simulink model "src_2022b"  (R2022b)
settings: Solver=VariableStepAuto  StartTime=0.0  StopTime=10.0  RelTol=1e-3
libraries: simulink x2, dspsrcs4 x1
settings Model: Creator=padlewsk  LastModifiedBy=padlewsk
settings OptimizationCC: ReuseModelBlockBuffer=on

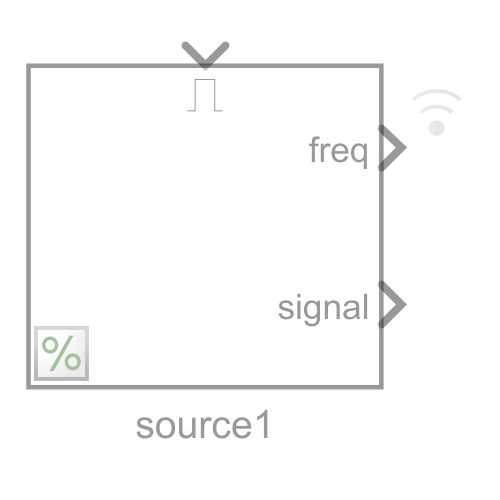
[thumbnail: Simulink's stored preview of the top-level diagram]
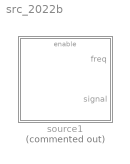
== system src_2022b ==
  source1 : Subsystem  Commented=on  TreatAsAtomicUnit=on

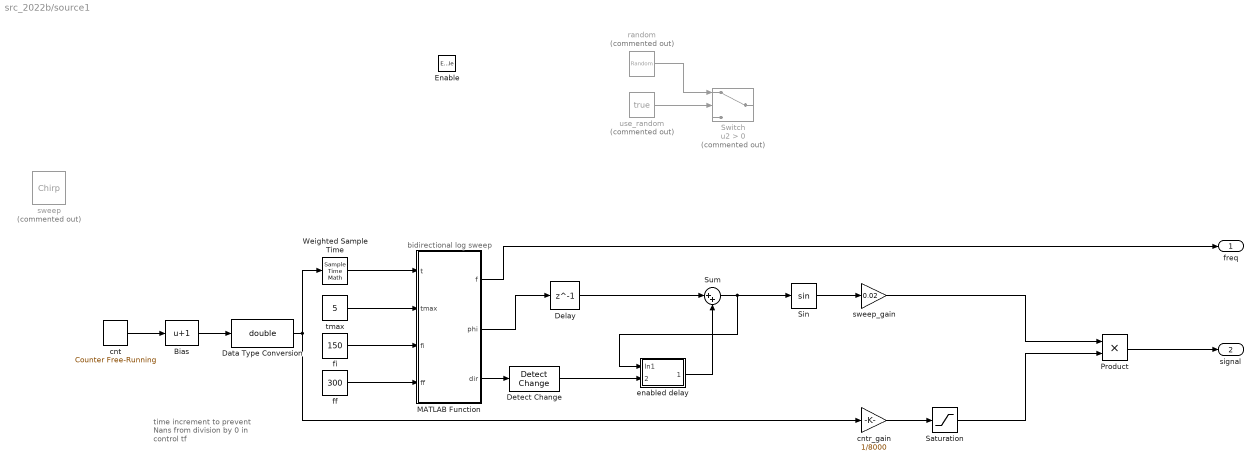
== system src_2022b/source1 ==
  note: bidirectional log sweep
  note: time increment to prevent Nans from division by 0 in control tf
  Enable : EnablePort  StatesWhenEnabling=reset
  Bias : Bias  Bias=1  SaturateOnIntegerOverflow=off
  Data Type Conversion : DataTypeConversion  OutDataTypeStr=double  SaturateOnIntegerOverflow=off  RndMeth=Floor
  Delay : Delay  DelayLength=1
  Detect Change : simulink/Logic and Bit Operations/Detect Change  vinit=false  OutDataTypeStr=boolean
  MATLAB Function : MATLAB Function  TreatAsAtomicUnit=on
  Product : Product
  Saturation : Saturate  UpperLimit=1  LowerLimit=0
  Sin : Trigonometry
  Sum : Sum  Inputs=|++
  Switch : Switch  Commented=on  Criteria=u2 > Threshold  SaturateOnIntegerOverflow=off  InputSameDT=off
  Weighted Sample Time : SampleTimeMath  TsampMathOp=*
  cnt : simulink/Sources/Counter Free-Running  NumBits=32  tsamp=-1
  cntr_gain : Gain  Gain=1/8000  ParamDataTypeStr=double
  enabled delay : Subsystem
  ff : Constant  Value=300
  fi : Constant  Value=150
  random : RandomNumber  Commented=on  Variance=0.5  SampleTime=3.5e-05
  sweep : dspsrcs4/Chirp  Commented=on  sweep=Logarithmic  mode=Bidirectional  f0=150  f1=1200  t1=10  Tsweep=20  phase=0  Ts=3.5e-05  spf=1  datatype=Double  OutputFrames=off
  sweep_gain : Gain  Gain=0.02
  tmax : Constant  Value=5
  use_random : Constant  Commented=on  Value=true  SampleTime=-1
  freq : Outport  OutputWhenDisabled=reset  InitialOutput=0  VectorParamsAs1DForOutWhenUnconnected=off
  signal : Outport  Port=2  OutputWhenDisabled=reset  InitialOutput=0  VectorParamsAs1DForOutWhenUnconnected=off
  wires:
  use_random/1 -> Switch/2
  random/1 -> Switch/1
  sweep_gain/1 -> Product/1
  cntr_gain/1 -> Saturation/1
  Product/1 -> signal/1
  MATLAB Function/2(phi) -> Delay/1
  Saturation/1 -> Product/2
  Weighted Sample Time/1 -> MATLAB Function/1(t)
  Data Type Conversion/1 -> cntr_gain/1, Weighted Sample Time/1
  MATLAB Function/1(f) -> freq/1
  Sin/1 -> sweep_gain/1
  MATLAB Function/3(dir) -> Detect Change/1
  Detect Change/1 -> enabled delay/2(enable)
  Delay/1 -> Sum/1
  enabled delay/1(Out1) -> Sum/2
  Sum/1 -> enabled delay/1(In1), Sin/1
  cnt/1 -> Bias/1
  Bias/1 -> Data Type Conversion/1
  ff/1 -> MATLAB Function/4(ff)
  tmax/1 -> MATLAB Function/2(tmax)
  fi/1 -> MATLAB Function/3(fi)

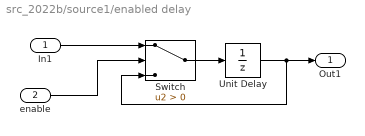
== system src_2022b/source1/enabled delay ==
  In1 : Inport
  enable : Inport  Port=2
  Switch : Switch  Criteria=u2 > Threshold  SaturateOnIntegerOverflow=off  InputSameDT=off
  Unit Delay : UnitDelay  SampleTime=-1  HasFrameUpgradeWarning=on
  Out1 : Outport
  wires:
  Unit Delay/1 -> Switch/3, Out1/1
  Switch/1 -> Unit Delay/1
  In1/1 -> Switch/1
  enable/1 -> Switch/2

== matlab function src_2022b/source1/MATLAB Function ==
  data: f output; t input; tmax input; phi output; dir output; fi input; ff input
function [f, phi, dir] = fcn(t, tmax, fi, ff)
%tmax is the time at which the maximum frequency is reached

t = mod(t, 2*tmax);

if t < tmax
    % up
    dir = 1;
    
    
    % linear (CF wikipedia)
%     phi = 2*pi*(0.5*(ff - fi)*t^2/tmax + fi*t);
%     f = fi + (ff - fi)*t/tmax;
    
    % logarithmic %%% https://en.wikipedia.org/wiki/Chirp
    k = log((ff/fi)^(1/tmax));
    phi = 2*pi*fi*(exp(k*t) - 1)/k;
    f = fi*exp(k*t);
else
    % down
    dir = -1;
    
    
    % linear (CF wikipedia)
%     phi = 2*pi*(0.5*(fi - ff)*(t-tmax)^2/tmax + ff*(t-tmax)); % linear
%     f = ff + (fi - ff)*(t - tmax)/tmax;
    
    % logarithmic
    k = log((fi/ff)^(1/tmax));
    phi = 2*pi*ff*(exp(k*(t - tmax)) - 1)/k;
    f = ff*exp(k*(t-tmax));
end

phi = mod(phi, 2*pi);
